simulink model "MH_96"  (R2018b)
settings: Solver=ode4  StartTime=0.0  StopTime=STOP_TIME  FixedStep=0.01  RelTol=1e-3
values from neighbouring files (symbols this model uses):
  Aircraft = tf(-Mdelta/Ta*[Ta, 1], [1, 2*Chi_a*Omega_a, Omega_a^2])    [run_MH_96_model.m]
  BandPass = tf([2*chi*Wn_act, 0], [1, 2*chi*Wn_act, Wn_act^2])    [run_MH_96_model.m]
  Gamma = 40    [run_MH_96_model.m]
  Ka = 1    [run_MH_96_model.m]
  Kq0 = 1    [run_MH_96_model.m]
  Notch = tf([1, 0, (2*Wn_act)^2], [1, 2*chi*(2*Wn_act), (2*Wn_act)^2])    [run_MH_96_model.m]
  RefModel = tf(-1, [Tau, 1])    [run_MH_96_model.m]
  T = 0.01    [run_MH_96_model.m]
libraries: simulink x2
settings Model: Creator=Rodney  LastModifiedBy=Rodney

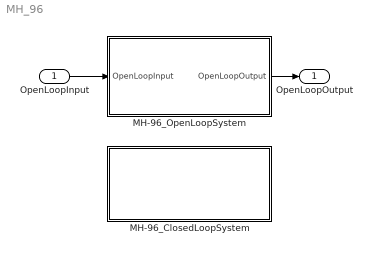
== system MH_96 ==
  OpenLoopInput : Inport
  MH-96_ClosedLoopSystem : Subsystem
  MH-96_OpenLoopSystem : Subsystem
  OpenLoopOutput : Outport
  wires:
  OpenLoopInput/1 -> MH-96_OpenLoopSystem/1(OpenLoopInput)
  MH-96_OpenLoopSystem/1(OpenLoopOutput) -> OpenLoopOutput/1

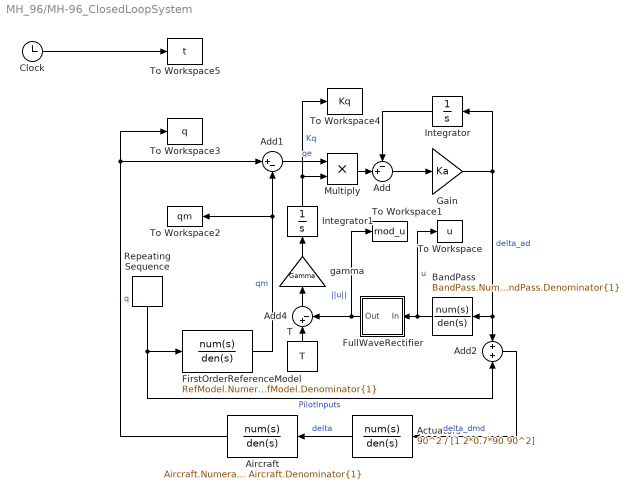
== system MH_96/MH-96_ClosedLoopSystem ==
  Actuators : TransferFcn  Numerator=90^2  Denominator=[1 2*0.7*90 90^2]
  Add : Sum  Inputs=-+|
  Add1 : Sum  Inputs=|+-
  Add2 : Sum  Inputs=+|+
  Add4 : Sum  Inputs=|+-
  Aircraft : TransferFcn  Numerator=Aircraft.Numerator{1}  Denominator=Aircraft.Denominator{1}
  BandPass : TransferFcn  Numerator=BandPass.Numerator{1}  Denominator=BandPass.Denominator{1}
  Clock : Clock
      settings: Decimation=100
  FirstOrderReferenceModel : TransferFcn  Numerator=RefModel.Numerator{1}  Denominator=RefModel.Denominator{1}
  FullWaveRectifier : Subsystem
  Gain : Gain  Gain=Ka
  Integrator : Integrator
  Integrator1 : Integrator  InitialCondition=Kq0  LimitOutput=on  UpperSaturationLimit=100  LowerSaturationLimit=0.5
  Multiply : Product
  Repeating Sequence : simulink/Sources/Repeating Sequence  rep_seq_t=[0 2 5 5.02 10 12]  rep_seq_y="[0 1 1 -1 -1  0] * 0.1"
  T : Constant  Value=T
  To Workspace : ToWorkspace  VariableName=u  SampleTime=-1
  To Workspace1 : ToWorkspace  VariableName=mod_u  SampleTime=-1
  To Workspace2 : ToWorkspace  VariableName=qm  SampleTime=-1
  To Workspace3 : ToWorkspace  VariableName=q  SampleTime=-1
  To Workspace4 : ToWorkspace  VariableName=Kq  SampleTime=-1
  To Workspace5 : ToWorkspace  VariableName=t  SampleTime=-1
  gamma : Gain  Gain=Gamma
  wires:
  Add/1 -> Gain/1
  Add2/1 -> Actuators/1  "delta_dmd"
  Actuators/1 -> Aircraft/1  "delta"
  Gain/1 -> Integrator/1, BandPass/1, Add2/1  "delta_ad"
  FirstOrderReferenceModel/1 -> Add1/2, To Workspace2/1  "qm"
  Repeating Sequence/1 -> FirstOrderReferenceModel/1, Add2/2  "PilotInputs"
  Integrator/1 -> Add/1
  Aircraft/1 -> To Workspace3/1, Add1/1  "q"
  BandPass/1 -> To Workspace/1, FullWaveRectifier/1(In)  "u"
  FullWaveRectifier/1(Out) -> To Workspace1/1, Add4/2  "||u||"
  T/1 -> Add4/1
  Add4/1 -> gamma/1
  Multiply/1 -> Add/2
  Add1/1 -> Multiply/1  "qe"
  Integrator1/1 -> To Workspace4/1, Multiply/2  "Kq"
  gamma/1 -> Integrator1/1
  Clock/1 -> To Workspace5/1

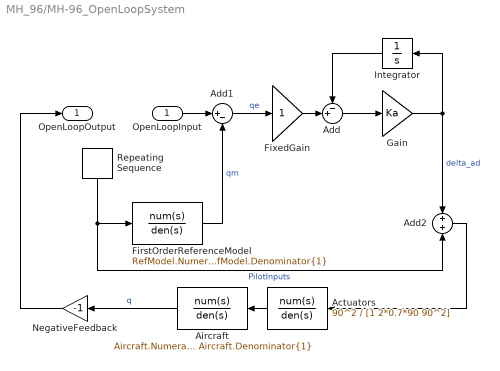
== system MH_96/MH-96_OpenLoopSystem ==
  OpenLoopInput : Inport
  Actuators : TransferFcn  Numerator=90^2  Denominator=[1 2*0.7*90 90^2]
  Add : Sum  Inputs=-+|
  Add1 : Sum  Inputs=|+-
  Add2 : Sum  Inputs=+|+
  Aircraft : TransferFcn  Numerator=Aircraft.Numerator{1}  Denominator=Aircraft.Denominator{1}
  FirstOrderReferenceModel : TransferFcn  Numerator=RefModel.Numerator{1}  Denominator=RefModel.Denominator{1}
  FixedGain : Gain
  Gain : Gain  Gain=Ka
  Integrator : Integrator
  NegativeFeedback : Gain  Gain=-1
  Repeating Sequence : simulink/Sources/Repeating Sequence  rep_seq_t=[0 2 5 5.02 10 12]  rep_seq_y="[0 1 1 -1 -1  0] * 0.1"
  OpenLoopOutput : Outport
  wires:
  Add1/1 -> FixedGain/1  "qe"
  FixedGain/1 -> Add/2
  Aircraft/1 -> NegativeFeedback/1  "q"
  Integrator/1 -> Add/1
  Repeating Sequence/1 -> Add2/2, FirstOrderReferenceModel/1  "PilotInputs"
  FirstOrderReferenceModel/1 -> Add1/2  "qm"
  Gain/1 -> Add2/1, Integrator/1  "delta_ad"
  Actuators/1 -> Aircraft/1
  Add2/1 -> Actuators/1
  Add/1 -> Gain/1
  OpenLoopInput/1 -> Add1/1
  NegativeFeedback/1 -> OpenLoopOutput/1

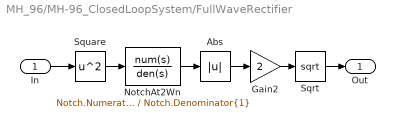
== system MH_96/MH-96_ClosedLoopSystem/FullWaveRectifier ==
  In : Inport
  Abs : Abs
  Gain2 : Gain  Gain=2
  NotchAt2Wn : TransferFcn  Numerator=Notch.Numerator{1}  Denominator=Notch.Denominator{1}
  Sqrt : Sqrt  SaturateOnIntegerOverflow=on
  Square : Math  Operator=square  SaturateOnIntegerOverflow=on
  Out : Outport
  wires:
  NotchAt2Wn/1 -> Abs/1
  Gain2/1 -> Sqrt/1
  In/1 -> Square/1
  Sqrt/1 -> Out/1
  Square/1 -> NotchAt2Wn/1
  Abs/1 -> Gain2/1
